simulink model "BitwiseOperator_TestGen4"  (R2017b)
settings: Solver=FixedStepDiscrete  StartTime=0.0  StopTime=10.0  RelTol=1e-3
undefined symbols (not defined in the file): Block_TestLib, reset
libraries: simulink x1
settings Model: Creator=hbourbou  LastModifiedBy=hbourbou
settings DebuggingCC: ParameterOverflowMsg=none

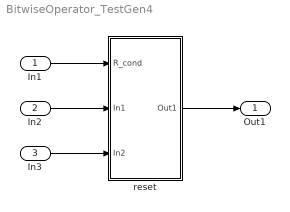
== system BitwiseOperator_TestGen4 ==
  In1 : Inport
  In2 : Inport  Port=2
  In3 : Inport  Port=3
  reset : Subsystem  AncestorBlock=Block_TestLib/reset
  Out1 : Outport
  wires:
  In1/1 -> reset/1(R_cond)
  In2/1 -> reset/2(In1)
  In3/1 -> reset/3(In2)
  reset/1(Out1) -> Out1/1

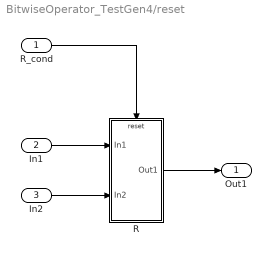
== system BitwiseOperator_TestGen4/reset ==
  R_cond : Inport  OutDataTypeStr=boolean
  In1 : Inport  Port=2
  In2 : Inport  Port=3
  R : Subsystem  TreatAsAtomicUnit=on
  Out1 : Outport
  wires:
  R_cond/1 -> R/Reset
  In1/1 -> R/1(In1)
  In2/1 -> R/2(In2)
  R/1(Out1) -> Out1/1

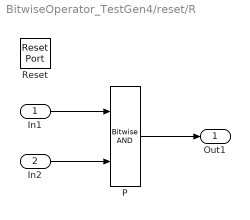
== system BitwiseOperator_TestGen4/reset/R ==
  In1 : Inport  OutDataTypeStr=uint16  PortDimensions=1
  In2 : Inport  Port=2
  Reset : ResetPort  DisableCoverage=on
  P : simulink/Logic and Bit Operations/Bitwise Operator  logicop=AND  UseBitMask=off  NumInputPorts=2  BitMask=bin2dec('11011001')  BitMaskRealWorld=Stored Integer
  Out1 : Outport
  wires:
  In1/1 -> P/1
  In2/1 -> P/2
  P/1 -> Out1/1
